simulink model "hybrid_powertrain_model"  (R2024b)
settings: Solver=VariableStepAuto  StartTime=0.0  StopTime=4800  MaxStep=0.5  RelTol=1e-3
values from neighbouring files (symbols this model uses):
  A = 2.08    [control_init.m]
  Cd = 0.4    [control_init.m]
  eta_gen = 0.87    [control_init.m]
  eta_mot = 0.88    [control_init.m]
  F_grade = m * g * sin(theta)    [control_init.m]
  F_rolling = Crr * m * g    (= 80.9325)    [control_init.m]
  m = 550    [control_init.m]
  P_apu_optimal_full = 1500    [control_init.m]
  Q_capacity = 31.25 * 3600    (= 112500)    [control_init.m]
  R_internal = 0.05    [control_init.m]
  rho = 1.18    [control_init.m]
  soc_breakpoints = [0.0, 0.1, 0.2, 0.3, 0.4, 0.5, 0.6, 0.7, 0.8, 0.9, 1.0]    [control_init.m]
  soc_high_threshold = 0.80    (= 0.8)    [control_init.m]
  soc_initial = 0.40    (= 0.4)    [control_init.m]
  soc_low_threshold = 0.30    (= 0.3)    [control_init.m]
  voc_values = [40.0, 42.5, 44.0, 45.5, 46.5, 47.5, 48.5, 49.5, 51.0, 52.5, 54.0]    [control_init.m]
settings Model: Creator=malit  LastModifiedBy=malit

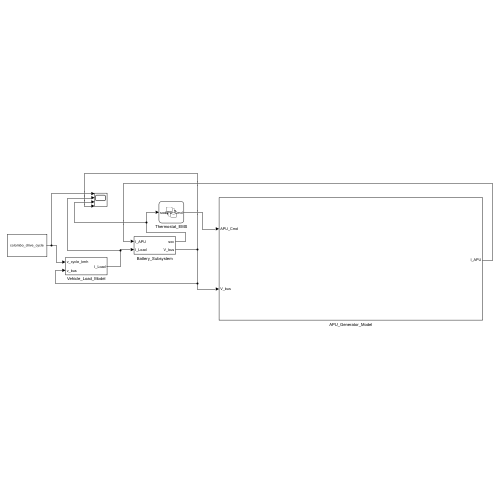
[thumbnail: Simulink's stored preview of the top-level diagram]
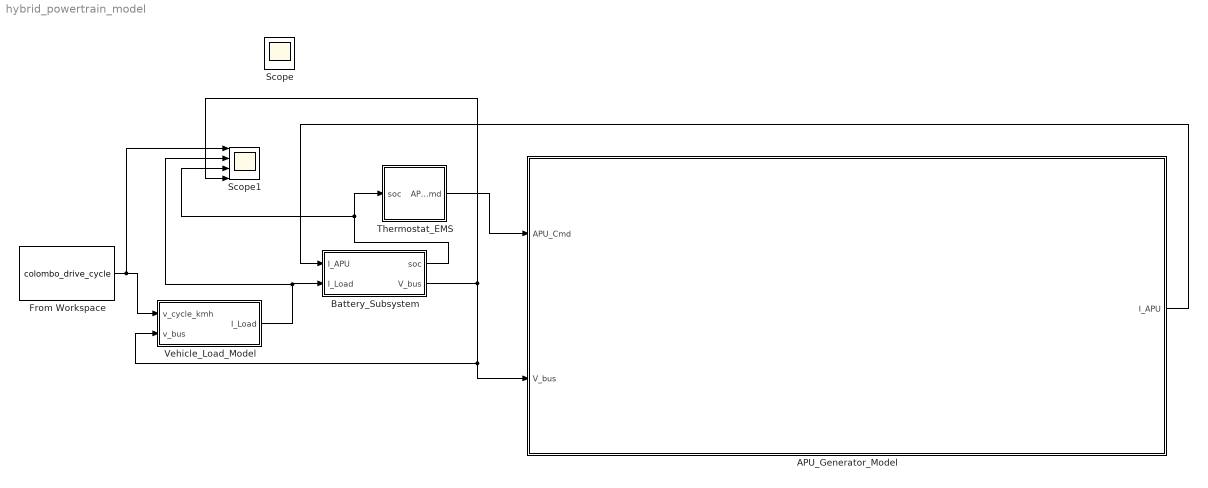
== system hybrid_powertrain_model ==
  APU_Generator_Model : Subsystem
  Battery_Subsystem : Subsystem
  From Workspace : FromWorkspace  VariableName=colombo_drive_cycle
  Scope1 : Scope  NumInputPorts=4
  Thermostat_EMS : Stateflow chart  TreatAsAtomicUnit=on
  Vehicle_Load_Model : Subsystem
  Scope : Scope
  wires:
  Thermostat_EMS/1(APU_Cmd) -> APU_Generator_Model/1(APU_Cmd)
  Battery_Subsystem/2(V_bus) -> Scope1/4, APU_Generator_Model/2(V_bus), Vehicle_Load_Model/2(v_bus)
  APU_Generator_Model/1(I_APU) -> Battery_Subsystem/1(I_APU)
  Battery_Subsystem/1(soc) -> Scope1/3, Thermostat_EMS/1(soc)
  From Workspace/1 -> Scope1/1, Vehicle_Load_Model/1(v_cycle_kmh)
  Vehicle_Load_Model/1(I_Load) -> Scope1/2, Battery_Subsystem/2(I_Load)

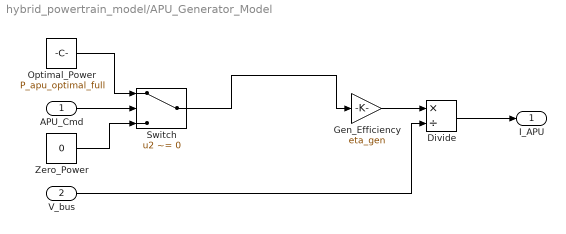
== system hybrid_powertrain_model/APU_Generator_Model ==
  APU_Cmd : Inport
  V_bus : Inport  Port=2
  Divide : Product  Inputs=*/
  Gen_Efficiency : Gain  Gain=eta_gen
  Optimal_Power : Constant  Value=P_apu_optimal_full
  Switch : Switch  Criteria=u2 ~= 0  Threshold=P_apu_optimal_full  SaturateOnIntegerOverflow=off  InputSameDT=off
  Zero_Power : Constant  Value=0
  I_APU : Outport
  wires:
  Switch/1 -> Gen_Efficiency/1
  APU_Cmd/1 -> Switch/2
  V_bus/1 -> Divide/2
  Divide/1 -> I_APU/1
  Zero_Power/1 -> Switch/3
  Optimal_Power/1 -> Switch/1
  Gen_Efficiency/1 -> Divide/1

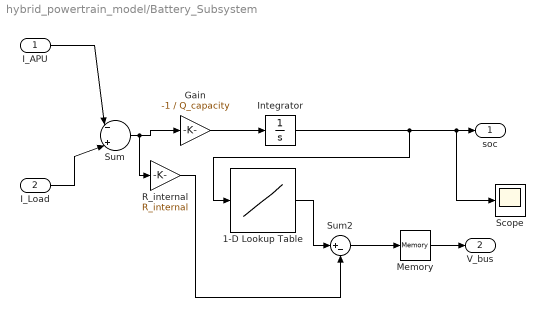
== system hybrid_powertrain_model/Battery_Subsystem ==
  I_APU : Inport
  I_Load : Inport  Port=2
  1-D Lookup Table : Lookup_n-D  NumberOfTableDimensions=1  BreakpointsForDimension1=soc_breakpoints  Table=voc_values  InternalRulePriority=Speed  RndMeth=Simplest
  Gain : Gain  Gain=-1 / Q_capacity
  Integrator : Integrator  InitialCondition=soc_initial
  Memory : Memory  InitialCondition=45.5
  R_internal : Gain  Gain=R_internal
  Scope : Scope
  Sum : Sum  Inputs=|-|+|
  Sum2 : Sum  Inputs=|+-
  soc : Outport
  V_bus : Outport  Port=2
  wires:
  I_APU/1 -> Sum/1
  I_Load/1 -> Sum/2
  Sum/1 -> R_internal/1, Gain/1
  Gain/1 -> Integrator/1
  Integrator/1 -> 1-D Lookup Table/1, Scope/1, soc/1
  R_internal/1 -> Sum2/2
  1-D Lookup Table/1 -> Sum2/1
  Sum2/1 -> Memory/1
  Memory/1 -> V_bus/1

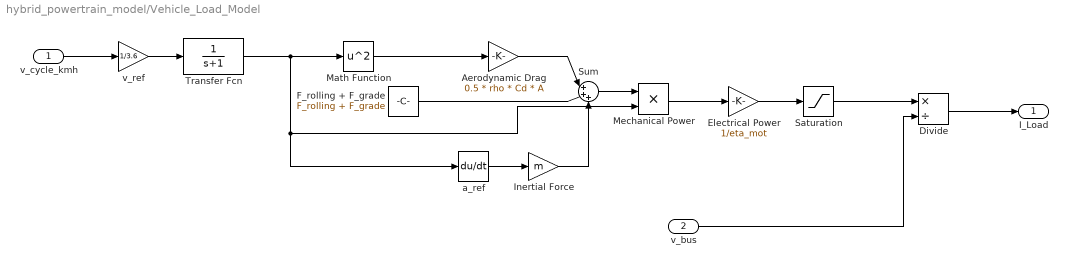
== system hybrid_powertrain_model/Vehicle_Load_Model ==
  v_cycle_kmh : Inport
  v_bus : Inport  Port=2
  Aerodynamic Drag : Gain  Gain=0.5 * rho * Cd * A
  Divide : Product  Inputs=*/
  Electrical Power : Gain  Gain=1/eta_mot
  F_rolling + F_grade : Constant  Value=F_rolling + F_grade
  Inertial Force : Gain  Gain=m
  Math Function : Math  Operator=square
  Mechanical Power : Product
  Saturation : Saturate  UpperLimit=inf  LowerLimit=0
  Sum : Sum  Inputs=|+++
  Transfer Fcn : TransferFcn  Denominator=[1 1]
  a_ref : Derivative
  v_ref : Gain  Gain=1/3.6
  I_Load : Outport
  wires:
  v_cycle_kmh/1 -> v_ref/1
  Math Function/1 -> Aerodynamic Drag/1
  a_ref/1 -> Inertial Force/1
  Aerodynamic Drag/1 -> Sum/1
  F_rolling + F_grade/1 -> Sum/2
  Inertial Force/1 -> Sum/3
  Sum/1 -> Mechanical Power/1
  Mechanical Power/1 -> Electrical Power/1
  v_bus/1 -> Divide/2
  Divide/1 -> I_Load/1
  Electrical Power/1 -> Saturation/1
  Saturation/1 -> Divide/1
  v_ref/1 -> Transfer Fcn/1
  Transfer Fcn/1 -> Mechanical Power/2, a_ref/1, Math Function/1

== stateflow chart hybrid_powertrain_model/Thermostat_EMS ==
  state ENGINE_OFF
    entry: APU_Cmd = false;
  state ENGINE_ON
    entry: APU_Cmd = true;
  (default) -> ENGINE_OFF
  ENGINE_OFF -> ENGINE_ON : [soc <= soc_low_threshold]
  ENGINE_ON -> ENGINE_OFF : [soc >= soc_high_threshold]
  data: soc input; APU_Cmd output; soc_low_threshold parameter; soc_high_threshold parameter
